simulink model "simulink_finance"  (R2021b)
settings: Solver=VariableStepAuto  StartTime=0.0  StopTime=1461  RelTol=1e-3
libraries: simulink x1
settings Model: Creator=maddi  LastModifiedBy=CHRIS KARATZIAS

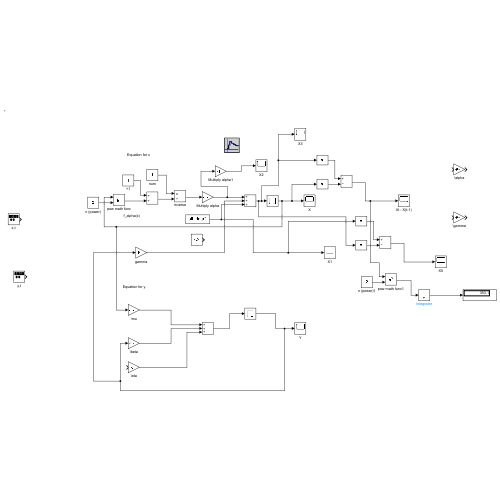
[thumbnail: Simulink's stored preview of the top-level diagram]
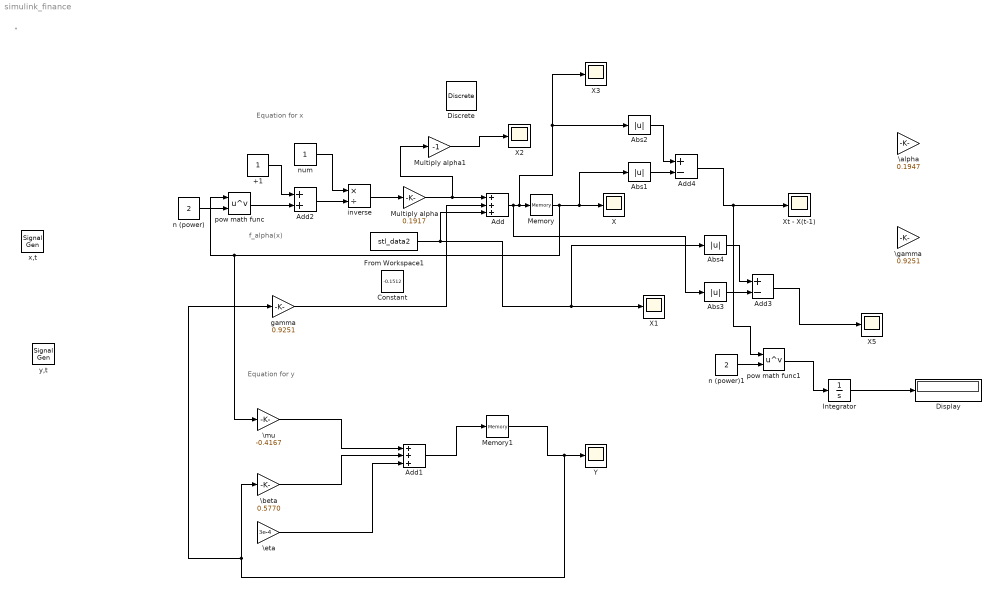
== system simulink_finance ==
  note: "
  note: Equation for y
  note: Equation for x
  note: f_alpha(x)
  +1 : Constant
  Abs{1..4} (4 alike) : Abs
  Add : Sum  Inputs=+++
  Add1 : Sum  Inputs=+++
  Add2 : Sum
  Add3 : Sum  Inputs=+-
  Add4 : Sum  Inputs=+-
  Constant : Constant  Value=-0.1512
  Discrete : simulink/Discrete  SystemSampleTime=-1  VariantActivationTime=update diagram  Latency=0  AutoFrameSizeCalculation=off
      settings: SourceProductBaseCode=SL
  Display : Display
  From Workspace1 : FromWorkspace  VariableName=stl_data2  SampleTime=1
  Integrator : Integrator
  Memory : Memory  InitialCondition=1
  Memory1 : Memory  InitialCondition=1
  Multiply alpha : Gain  Gain=0.1917
  Multiply alpha1 : Gain  Gain=-1
  X{,1..3,5} (5 alike) : Scope
  Xt - X(t-1) : Scope
  Y : Scope
  \alpha : Gain  Gain=0.1947
  \beta : Gain  Gain=0.5770
  \eta : Gain  Gain=3e-4
  \gamma : Gain  Gain=0.9251
  \mu : Gain  Gain=-0.4167
  gamma : Gain  Gain=0.9251
  inverse : Product  Inputs=*/
  n (power) : Constant  Value=2
  n (power)1 : Constant  Value=2
  num : Constant
  pow math func : Math  Operator=pow  SaturateOnIntegerOverflow=on
  pow math func1 : Math  Operator=pow  SaturateOnIntegerOverflow=on
  x,t : SignalGenerator  WaveForm=random  Units=rad/sec
  y,t : SignalGenerator  WaveForm=random  Units=rad/sec
  wires:
  n (power)/1 -> pow math func/2
  pow math func/1 -> Add2/2
  num/1 -> inverse/1
  Add2/1 -> inverse/2
  inverse/1 -> Multiply alpha/1
  gamma/1 -> Add/2
  \mu/1 -> Add1/1
  \beta/1 -> Add1/2
  \eta/1 -> Add1/3
  +1/1 -> Add2/1
  Memory/1 -> \mu/1, pow math func/1, Abs1/1, X/1
  Add1/1 -> Memory1/1
  Memory1/1 -> \beta/1, gamma/1, Y/1
  From Workspace1/1 -> Abs4/1, X1/1, Add/3
  Multiply alpha/1 -> Multiply alpha1/1, Add/1
  Multiply alpha1/1 -> X2/1
  Abs2/1 -> Add4/1
  Add4/1 -> Xt - X(t-1)/1, pow math func1/1
  Abs1/1 -> Add4/2
  Abs4/1 -> Add3/1
  Abs3/1 -> Add3/2
  n (power)1/1 -> pow math func1/2
  Add3/1 -> X5/1
  pow math func1/1 -> Integrator/1
  Integrator/1 -> Display/1
  Add/1 -> Abs3/1, Abs2/1, X3/1, Memory/1
